simulink model "example_Hydraulic_MixingValvePt1"  (R2018b)
settings: Solver=ode45  StartTime=0.0  StopTime=400  RelTol=1e-3
undefined symbols (not defined in the file): linear, path_carnot
libraries: carnot x14, simulink x4, simulink_extras x1
settings Model: Creator=drhf  LastModifiedBy=P41573
settings SolverCC: ZeroCrossAlgorithm=Adaptive
settings DebuggingCC: MaxConsecutiveZCsMsg=none  IgnoredZcDiagnostic=none
settings SFSimCC: SimUseLocalCustomCode=off
settings RTWCC: RTWUseLocalCustomCode=off
settings CodeAppCC: StateflowObjectComments=on

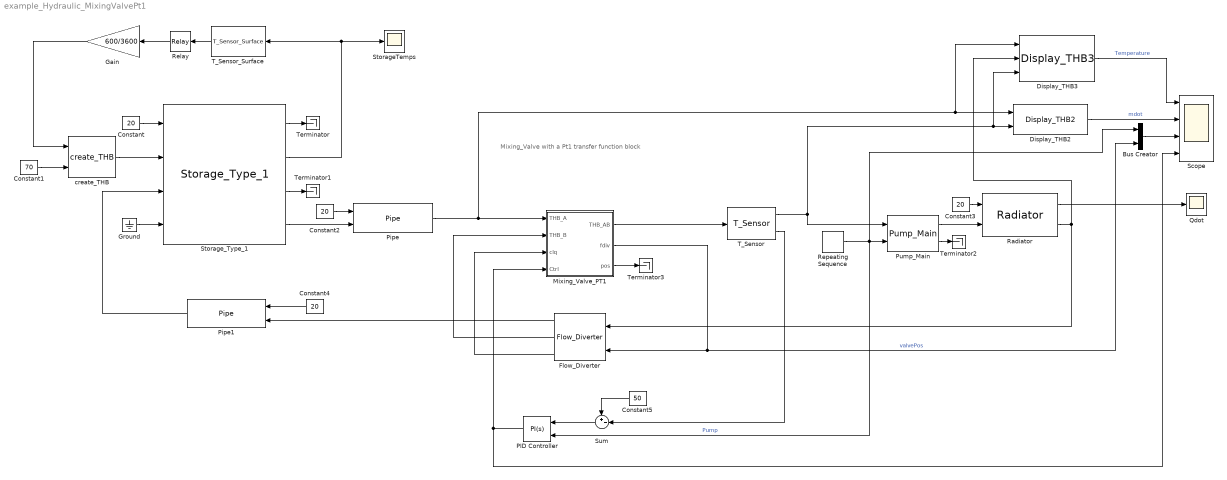
== system example_Hydraulic_MixingValvePt1 ==
  note: Mixing_Valve with a Pt1 transfer function block
  Bus Creator : BusCreator  Inputs=2
  Constant{,2..4} (4 alike) : Constant  Value=20
  Constant1 : Constant  Value=70
  Constant5 : Constant  Value=50
  Display_THB2 : carnot/Outputs/Display_THB2  t=off  m=on  p=off  id=off  mix=off  d=off
      settings: SourceProductName=Carnot
  Display_THB3 : carnot/Outputs/Display_THB3  t=on  m=off  p=off  id=off  mix=off  d=off
      settings: SourceProductName=Carnot
  Flow_Diverter : carnot/Hydraulics/Flow_Diverter
      settings: SourceProductName=Carnot
  Gain : Gain  Gain=600/3600
  Ground : Ground
  Mixing_Valve_PT1 : Subsystem  mask(Mixing Valve){Art_A=linear, Art_B=linear, kvs=1.6, psi_0=0.01, dt_V=30, t_fdiv=1}
      mask prompts: Art_A "Valve characteristic A->AB"; Art_B "Valve characteristic B->AB"; kvs "Kvs: flow coefficient of the open valve in m³/h"; psi_0 "Psi_0: relative flow coefficient Kv/Kvs of the closed valve"; dt_V "Valve running time in s"; t_fdiv "Time constant for fdiv in s"
      mask help:
      | Mixes two massflows and calculates the pressure drop of the branches. The new temperature is calculated by an energy balance. The output f_div may be fed back to the corresponding flow diverter upwards in flowdirection.
      | This model uses a Memory block to break an algebraic loop. Avoid using the variable-step solver ode15s or ode113 (see block help for details).
      mask Help: web(fullfile(path_carnot('help'),'Mixing_Valve.html'),'-helpbrowser')
      mask TypeOptions Art_A: Valve_A/vtyp
      mask TypeOptions Art_B: Valve_B/vtyp
      mask TypeOptions kvs: Valve_A/kvs | Valve_B/kvs
      mask TypeOptions psi_0: Valve_A/psi_0 | Valve_B/psi_0
      mask TypeOptions dt_V: Valve_A/dt_V | Valve_B/dt_V
      mask TypeOptions t_fdiv: PT1_for_fdiv/t_fdiv
      mask Display:
      | plot(-20,-5,110,90,...
      |     [20 50 20 20],[20 30 40 20],...
      |     [50 80 80 50],[30 20 40 30],...
      |     [50 40 60 50],[30 10 10 30],...
      |     [50,50],[45,30],...
      |     [40,30,30,40,60,70,70,60,40],[45,50,60,65,65,60,50,45,45],...
      |     [60,60,50,40,40],[50,60,55,60,50])
  PID Controller : simulink/Continuous/PID Controller  Controller=PI  Form=Parallel  TimeDomain=Continuous-time  SampleTime=-1  IntegratorMethod=Forward Euler  FilterMethod=Forward Euler  ControllerParametersSource=internal  P=0.05  I=0.001  D=0  UseFilter=on  N=100  TunerSelectOption=Transfer Function Based (PID Tuner App)  InitialConditionSource=internal  InitialConditionForIntegrator=0.5  InitialConditionForFilter=0  DifferentiatorICPrevScaledInput=0  ExternalReset=rising  TrackingMode=off  Kt=1  LimitOutput=on  UpperSaturationLimit=1  LowerSaturationLimit=0  LinearizeAsGain=on  AntiWindupMode=clamping  Kb=1  POutMin=[]  POutMax=[]  IOutMin=[]  IOutMax=[]  DOutMin=[]  DOutMax=[]  NOutMin=[]  NOutMax=[]  SumOutMin=[]  SumOutMax=[]  SaturationOutMin=[]  SaturationOutMax=[]  PParamMin=[]  PParamMax=[]  IParamMin=[]  IParamMax=[]  DParamMin=[]  DParamMax=[]  NParamMin=[]  NParamMax=[]  KbParamMin=[]  KbParamMax=[]  KtParamMin=[]  KtParamMax=[]  KbOutMin=[]  KbOutMax=[]  KtOutMin=[]  KtOutMax=[]  IntegratorOutMin=[]  IntegratorOutMax=[]  FilterOutMin=[]  FilterOutMax=[]  SumI1OutMin=[]  SumI1OutMax=[]  SumI2OutMin=[]  SumI2OutMax=[]  SumI3OutMin=[]  SumI3OutMax=[]  SumI4OutMin=[]  SumI4OutMax=[]  SumDOutMin=[]  SumDOutMax=[]  DifferentiatorOutMin=[]  DifferentiatorOutMax=[]  FilterDiffOutCoefMin=[]  FilterDiffOutCoefMax=[]  ReciprocalOutMin=[]  ReciprocalOutMax=[]  SumDenOutMin=[]  SumDenOutMax=[]  SumNumOutMin=[]  SumNumOutMax=[]  DivideOutMin=[]  DivideOutMax=[]  IntegratorContinuousStateAttributes=''  IntegratorStateMustResolveToSignalObject=off  IntegratorRTWStateStorageClass=Auto  FilterContinuousStateAttributes=''  FilterStateMustResolveToSignalObject=off  FilterRTWStateStorageClass=Auto  ParallelPVariant=InternalParameters  IdealPVariant=Disabled  IVariant=InternalParameters  DVariant=Disabled  IntegratorVariant=Continuous  SatVariant=Enabled  AWVariant=ContClampingParallel  PCopyVariant=Disabled  TRVariant=Disabled  FdbkBlocksVariant=Forward  IdealPFdbkVariant=Disabled  SatFdbkVariant=Disabled  DerivativeFilterVariant=Disabled  NVariant=Disabled  NCopyVariant=Disabled_SignalSpec  FilterICVariant=Disabled  IntegratorICVariant=InternalICs  ExternalResetVariant=ExternalReset  TRSumVariant=Passthrough  SumFdbkVariant=Disabled  SumVariant=Sum_PI
  Pipe : carnot/Hydraulics/Pipe  dia=0.025  len=10  hgt=0  uloss=100/20/10  cond=0  cwall=1000  t0=20  lin=10  qua=10  nodes=10
      settings: SourceProductName=Carnot
  Pipe1 : carnot/Hydraulics/Pipe  dia=0.025  len=10  hgt=0  uloss=100/20/10  cond=0  cwall=1000  t0=20  lin=10  qua=10  nodes=10
      settings: SourceProductName=Carnot
  Pump_Main : carnot/Hydraulics/Pump_Main  Tini=20  p0=3e5  IDpreset=pressure drop  fluid=Water  mix=0  mix2=0  mix3=0  t1=5  PathName=fullfile(path_carnot('libsl'), 'Hydraulics', 'Pump_Main', 'parameter_set')  FileName='Pump6m.mat'  userPath=off  userParam=off  a0=60000  a1=-43200  a2=0  dia=0.025  UA=1  mcp=4182  e0=50  e1=28.8  e2=-10.368
      settings: SourceProductName=Carnot
  Qdot : Scope
  Radiator : carnot/Source/Heat_Exchanger/Radiator  pnom=5000  dtnom=49.83  expo=1.3  mcap=5*4182  tini=20  lin=10  qua=10
      settings: SourceProductName=Carnot
  Relay : Relay  OnSwitchValue=70  OffSwitchValue=60  OnOutputValue=0  OffOutputValue=1
  Repeating Sequence : simulink/Sources/Repeating Sequence  rep_seq_t=[0 20 60 200]  rep_seq_y=[0 0 1 1]
  Scope : Scope  NumInputPorts=4
  StorageTemps : Scope
  Storage_Type_1 : carnot/Storage/Thermal/Storage_Type_1  t0=70  hgt=1.7684  stgtype=1  tini=[70 70 70 70 70 70 70 70 70 70]  mpts=[1 2 3 4 5 6 7 8 9 10]  PathName=fullfile(path_carnot('libsl'),'Storage','Thermal','Storage_Type_1','parameter_set')  FileName='StorageType1_500_L.mat'  userPath=off  userParam=off  uwall=1  ubot=1  utop=1  axcond=1  volume=0.5  dia=0.6  standing=standing cylinder  nodes=10  mpoints=10  Tsensor=0.5  pipe1inlet=1  pipe1outlet=0  pipe1dia=0.03  pipe2inlet=0  pipe2outlet=1  pipe2dia=0.03  heater1start=0.6  heater1end=0.65
      settings: SourceProductName=Carnot
  Sum : Sum  Inputs=+-|
  T_Sensor : carnot/Control/T_Sensor  tc=10  t0=20
      settings: SourceProductName=Carnot
  T_Sensor_Surface : carnot/Control/T_Sensor_Surface  pos=0.5  tdel=1  t0=70
      settings: SourceProductName=Carnot
  Terminator{,1..3} (4 alike) : Terminator
  create_THB : carnot/Source/Simple/create_THB  p=1e5  fluid=Water  mix=0  mix2=0  mix3=0  dia=0  hgt=0  mID=No Pressure Drop
      settings: SourceProductName=Carnot
  wires:
  Constant/1 -> Storage_Type_1/1
  Storage_Type_1/1 -> Terminator/1
  Storage_Type_1/3 -> Terminator1/1
  Storage_Type_1/2 -> T_Sensor_Surface/1, StorageTemps/1
  create_THB/1 -> Storage_Type_1/2
  Constant1/1 -> create_THB/2
  T_Sensor_Surface/1 -> Relay/1
  Relay/1 -> Gain/1
  Gain/1 -> create_THB/1
  Constant2/1 -> Pipe/1
  Pump_Main/2 -> Terminator2/1
  Pipe/1 -> Mixing_Valve_PT1/1(THB_A), Display_THB3/1, Display_THB2/1
  Repeating Sequence/1 -> Bus Creator/1, PID Controller/2, Pump_Main/2  "Pump"
  Pump_Main/1 -> Radiator/2
  Radiator/1 -> Qdot/1
  Radiator/2 -> Flow_Diverter/1, Display_THB3/2
  Constant3/1 -> Radiator/1
  Display_THB2/1 -> Scope/2  "mdot"
  Storage_Type_1/4 -> Pipe/2
  Constant4/1 -> Pipe1/1
  Pipe1/1 -> Storage_Type_1/3
  Flow_Diverter/1 -> Pipe1/2
  Flow_Diverter/2 -> Mixing_Valve_PT1/2(THB_B)
  Flow_Diverter/3 -> Mixing_Valve_PT1/3(clq)
  Mixing_Valve_PT1/2(fdiv) -> Bus Creator/2, Flow_Diverter/2  "valvePos"
  T_Sensor/1 -> Display_THB2/2, Display_THB3/3, Pump_Main/1
  Bus Creator/1 -> Scope/3
  Display_THB3/1 -> Scope/1  "Temperature"
  Sum/1 -> PID Controller/1
  Constant5/1 -> Sum/1
  T_Sensor/2 -> Sum/2
  Mixing_Valve_PT1/1(THB_AB) -> T_Sensor/1
  PID Controller/1 -> Mixing_Valve_PT1/4(Ctrl), Scope/4
  Mixing_Valve_PT1/3(pos) -> Terminator3/1
  Ground/1 -> Storage_Type_1/4

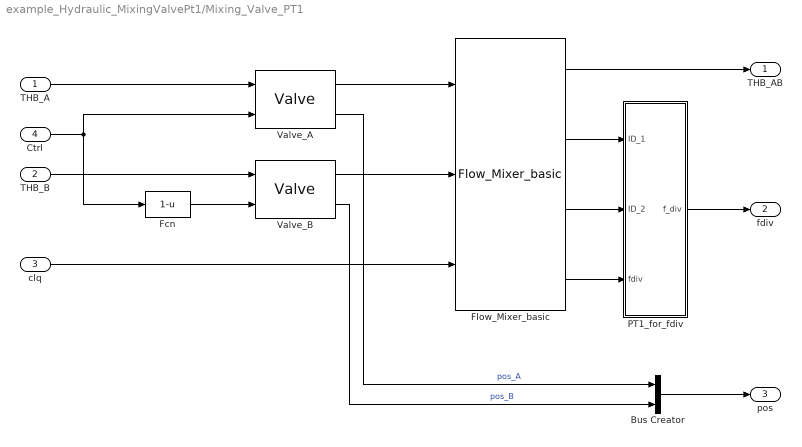
== system example_Hydraulic_MixingValvePt1/Mixing_Valve_PT1 ==
  THB_A : Inport
  THB_B : Inport  Port=2
  clq : Inport  Port=3
  Ctrl : Inport  Port=4
  Bus Creator : BusCreator  Inputs=2
  Fcn : Fcn  Expr=1-u
  Flow_Mixer_basic : carnot/Basic/Hydraulics/Flow_Mixer_basic
      settings: SourceProductName=Carnot
  PT1_for_fdiv : Subsystem  mask{t_fdiv=t_fdiv}
      mask prompts: t_fdiv "Time constant for fdiv in s"
  Valve_A : carnot/Hydraulics/Valve  vtyp=linear  psi_0=psi_0  kvs=kvs  dt_V=dt_V
      settings: SourceProductName=Carnot
  Valve_B : carnot/Hydraulics/Valve  vtyp=linear  psi_0=psi_0  kvs=kvs  dt_V=dt_V
      settings: SourceProductName=Carnot
  THB_AB : Outport
  fdiv : Outport  Port=2
  pos : Outport  Port=3
  wires:
  Fcn/1 -> Valve_B/2
  Valve_B/2 -> Bus Creator/2  "pos_B"
  Valve_A/2 -> Bus Creator/1  "pos_A"
  Bus Creator/1 -> pos/1
  Valve_B/1 -> Flow_Mixer_basic/2
  Ctrl/1 -> Valve_A/2, Fcn/1
  THB_B/1 -> Valve_B/1
  Valve_A/1 -> Flow_Mixer_basic/1
  clq/1 -> Flow_Mixer_basic/3
  PT1_for_fdiv/1(f_div) -> fdiv/1
  THB_A/1 -> Valve_A/1
  Flow_Mixer_basic/1 -> THB_AB/1
  Flow_Mixer_basic/2 -> PT1_for_fdiv/1(ID_1)
  Flow_Mixer_basic/3 -> PT1_for_fdiv/2(ID_2)
  Flow_Mixer_basic/4 -> PT1_for_fdiv/3(fdiv)

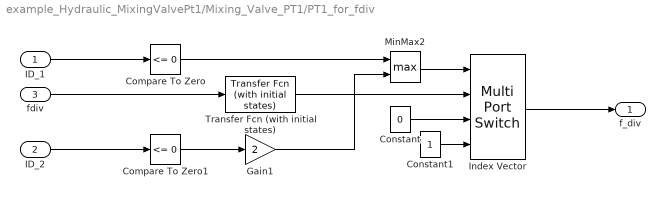
== system example_Hydraulic_MixingValvePt1/Mixing_Valve_PT1/PT1_for_fdiv ==
  ID_1 : Inport
  ID_2 : Inport  Port=2
  fdiv : Inport  Port=3
  Compare To Zero : simulink/Logic and Bit Operations/Compare To Zero  relop=<=  OutDataTypeStr=uint8
  Compare To Zero1 : simulink/Logic and Bit Operations/Compare To Zero  relop=<=  OutDataTypeStr=uint8
  Constant : Constant  Value=0
  Constant1 : Constant
  Gain1 : Gain  Gain=2
  Index Vector : MultiPortSwitch  DataPortOrder=Zero-based contiguous  zeroidx=on
  MinMax2 : MinMax  Function=max  Inputs=2
  Transfer Fcn (with initial states) : simulink_extras/Additional Linear/Transfer Fcn (with initial states)  N=[1]  D="[t_fdiv  1]"  X0=0.5*t_fdiv
  f_div : Outport
  wires:
  fdiv/1 -> Transfer Fcn (with initial states)/1
  Compare To Zero1/1 -> Gain1/1
  Compare To Zero/1 -> MinMax2/1
  MinMax2/1 -> Index Vector/1
  ID_1/1 -> Compare To Zero/1
  ID_2/1 -> Compare To Zero1/1
  Constant/1 -> Index Vector/3
  Transfer Fcn (with initial states)/1 -> Index Vector/2
  Constant1/1 -> Index Vector/4
  Gain1/1 -> MinMax2/2
  Index Vector/1 -> f_div/1
